simulink model "lab2_1"  (R2021b)
settings: Solver=VariableStepAuto  StartTime=0.0  StopTime=10.0  RelTol=1e-3
values from neighbouring files (symbols this model uses):
  g = 9.81    [lab2.m]
  km = 0.1    [lab2.m]
  La = 0.05    [lab2.m]
  M = 0.1    [lab2.m]
  Ra = 3    [lab2.m]
settings Model: Creator=jiayizhou  LastModifiedBy=zlt05
settings SolverCC: AlgebraicLoopSolver=TrustRegion
settings DebuggingCC: SFMachineParentedDataDiag=warning

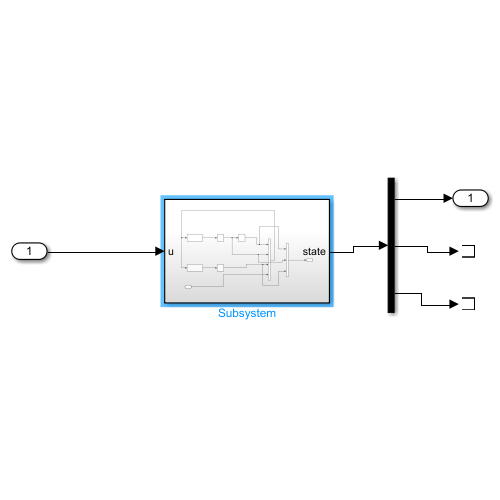
[thumbnail: Simulink's stored preview of the top-level diagram]
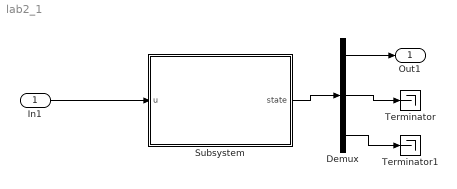
== system lab2_1 ==
  In1 : Inport  PortDimensions=1
  Demux : Demux  Outputs=3
  Subsystem : Subsystem
  Terminator : Terminator
  Terminator1 : Terminator
  Out1 : Outport
  wires:
  In1/1 -> Subsystem/1(u)
  Subsystem/1(state) -> Demux/1
  Demux/1 -> Out1/1
  Demux/2 -> Terminator/1
  Demux/3 -> Terminator1/1

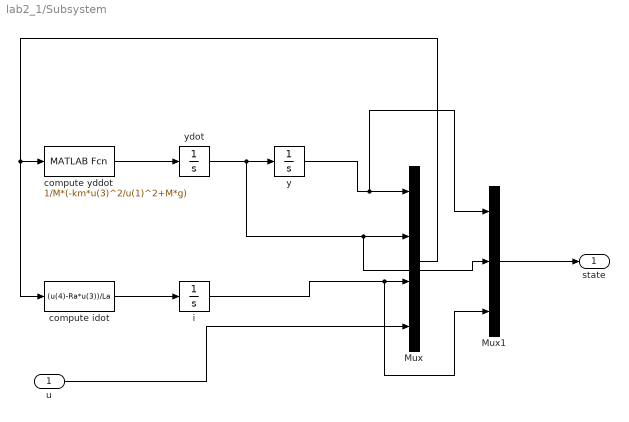
== system lab2_1/Subsystem ==
  u : Inport
  Mux : Mux
  Mux1 : Mux  Inputs=3
  compute idot : MATLABFcn  MATLABFcn=(u(4)-Ra*u(3))/La
  compute yddot : MATLABFcn  MATLABFcn=1/M*(-km*u(3)^2/u(1)^2+M*g)
  i : Integrator
  y : Integrator
  ydot : Integrator
  state : Outport
  wires:
  u/1 -> Mux/4
  Mux1/1 -> state/1
  i/1 -> Mux1/3, Mux/3
  compute idot/1 -> i/1
  compute yddot/1 -> ydot/1
  ydot/1 -> Mux1/2, Mux/2, y/1
  y/1 -> Mux/1, Mux1/1
  Mux/1 -> compute idot/1, compute yddot/1
